simulink model "trajectory_evaluator"  (R2016a)
settings: Solver=VariableStepAuto  StartTime=0.0  StopTime=30.0  RelTol=1e-3
settings Model: Creator=mgreiff  LastModifiedBy=mgreiff

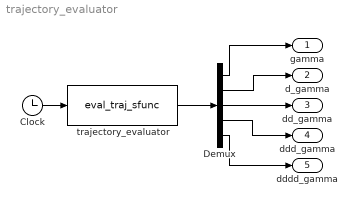
== system trajectory_evaluator ==
  Clock : Clock
  Demux : Demux  Outputs=[4,4,4,4,4]
  trajectory_evaluator : S-Function  FunctionName=eval_traj_sfunc  Parameters=trajectory  SFunctionDeploymentMode=off  EnableBusSupport=off
  gamma : Outport
  d_gamma : Outport  Port=2
  dd_gamma : Outport  Port=3
  ddd_gamma : Outport  Port=4
  dddd_gamma : Outport  Port=5
  wires:
  trajectory_evaluator/1 -> Demux/1
  Demux/3 -> dd_gamma/1
  Demux/4 -> ddd_gamma/1
  Demux/5 -> dddd_gamma/1
  Demux/2 -> d_gamma/1
  Demux/1 -> gamma/1
  Clock/1 -> trajectory_evaluator/1
